simulink model "class_6_simulink"  (R2023b)
settings: Solver=VariableStepAuto  StartTime=0.0  StopTime=10.0  RelTol=1e-3
values from neighbouring files (symbols this model uses):
  denp = [3 1]    [class_6.m]
  h = 6.5    [class_6.m]
  nump = 2    [class_6.m]
libraries: cstblocks x3
settings Model: Creator=klysm  LastModifiedBy=klysm

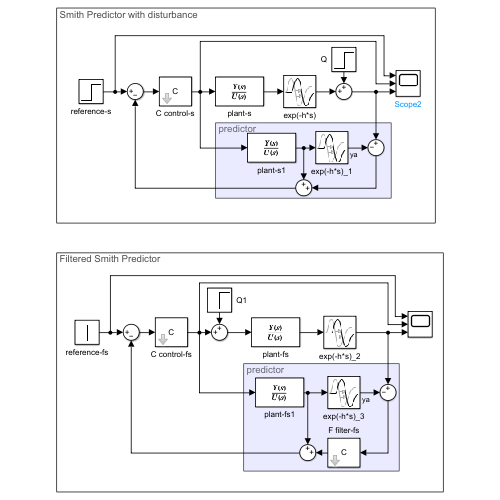
[thumbnail: Simulink's stored preview of the top-level diagram]
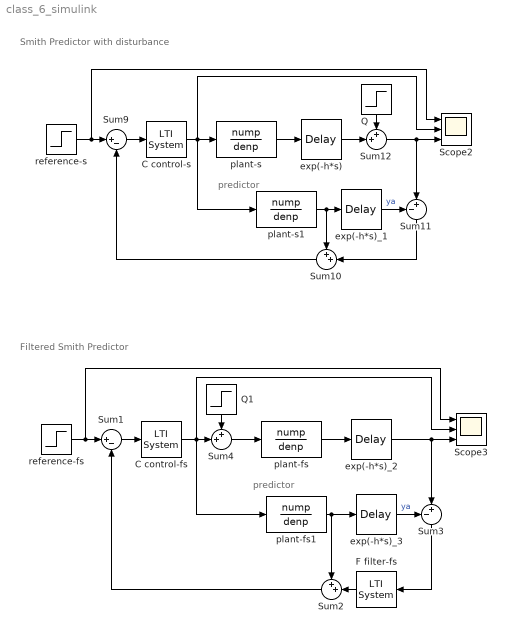
== system class_6_simulink ==
  note: Filtered Smith Predictor
  note: predictor
  note: Smith Predictor with disturbance
  note: predictor
  C control-fs : cstblocks/LTI System  sys=C  IC=[]  PadeOrder=0
  C control-s : cstblocks/LTI System  sys=C  IC=[]  PadeOrder=0
  F filter-fs : cstblocks/LTI System  sys=C  IC=[]  PadeOrder=0
  Q : Step  Time=8  SampleTime=0
  Q1 : Step  SampleTime=0
  Scope2 : Scope  NumInputPorts=3
  Scope3 : Scope  NumInputPorts=3
  Sum1 : Sum  Inputs=|+-
  Sum{2,4,10,12} (4 alike) : Sum  Inputs=++|
  Sum11 : Sum  Inputs=-+|
  Sum3 : Sum  Inputs=-+|
  Sum9 : Sum  Inputs=|+-
  exp(-h*s) : TransportDelay  DelayTime=h
  exp(-h*s)_1 : TransportDelay  DelayTime=h
  exp(-h*s)_2 : TransportDelay  DelayTime=h
  exp(-h*s)_3 : TransportDelay  DelayTime=h
  plant-fs : TransferFcn  Numerator=nump  Denominator=denp
  plant-fs1 : TransferFcn  Numerator=nump  Denominator=denp
  plant-s : TransferFcn  Numerator=nump  Denominator=denp
  plant-s1 : TransferFcn  Numerator=nump  Denominator=denp
  reference-fs : Step  SampleTime=0
  reference-s : Step  Time=0  SampleTime=0
  wires:
  Sum3/1 -> F filter-fs/1
  reference-fs/1 -> Scope3/1, Sum1/1
  plant-fs1/1 -> exp(-h*s)_3/1, Sum2/1
  plant-fs/1 -> exp(-h*s)_2/1
  Sum2/1 -> Sum1/2
  exp(-h*s)_3/1 -> Sum3/1  "ya"
  Sum4/1 -> plant-fs/1
  exp(-h*s)_2/1 -> Scope3/3, Sum3/2
  Sum1/1 -> C control-fs/1
  Q1/1 -> Sum4/1
  F filter-fs/1 -> Sum2/2
  plant-s/1 -> exp(-h*s)/1
  reference-s/1 -> Scope2/1, Sum9/1
  Sum12/1 -> Scope2/3, Sum11/2
  Sum10/1 -> Sum9/2
  Sum9/1 -> C control-s/1
  Q/1 -> Sum12/1
  C control-s/1 -> Scope2/2, plant-s/1, plant-s1/1
  exp(-h*s)_1/1 -> Sum11/1  "ya"
  plant-s1/1 -> Sum10/1, exp(-h*s)_1/1
  exp(-h*s)/1 -> Sum12/2
  Sum11/1 -> Sum10/2
  C control-fs/1 -> Scope3/2, Sum4/2, plant-fs1/1
